simulink model "Sample156"  (Simulink 7.6)
settings: Solver=ode45  StartTime=0.0  StopTime=10.0  RelTol=1e-3
undefined symbols (not defined in the file): randint
libraries: commdigbbndfm2 x2, simulink x1, dspsrcs4 x1, commblkcod2 x1
settings Model: Creator=zhangling  LastModifiedBy=zhangling

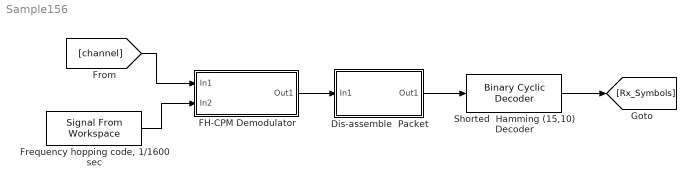
== system Sample156 ==
  Dis-assemble  Packet : Subsystem
  FH-CPM Demodulator : Subsystem
  "Frequency hopping code, 1/1600 sec" : dspsrcs4/Signal From Workspace  SystemSampleTime=-1  X=randint(1,100,78)  Ts=1/1600  nsamps=1  OutputAfterFinalValue=Cyclic repetition  ignoreOrWarnInputAndFrameLengths=off
  Shorted  Hamming (15,10) Decoder : commblkcod2/Binary Cyclic Decoder  SystemSampleTime=-1  n=7  p=4
  wires:
  [channel] -> FH-CPM Demodulator/1(In1)
  "Frequency hopping code, 1/1600 sec"/1 -> FH-CPM Demodulator/2(In2)
  Dis-assemble  Packet/1(Out1) -> Shorted  Hamming (15,10) Decoder/1
  FH-CPM Demodulator/1(Out1) -> Dis-assemble  Packet/1(In1)
  Shorted  Hamming (15,10) Decoder/1 -> [Rx_Symbols]

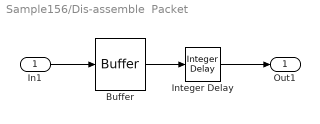
== system Sample156/Dis-assemble  Packet ==
  In1 : Inport
  Buffer : Buffer  N=15  TreatMby1Signals=One channel
  Integer Delay : simulink/Discrete/Integer Delay  NumDelays=10  vinit=0.0  samptime=-1
  Out1 : Outport
  wires:
  In1/1 -> Buffer/1
  Buffer/1 -> Integer Delay/1
  Integer Delay/1 -> Out1/1

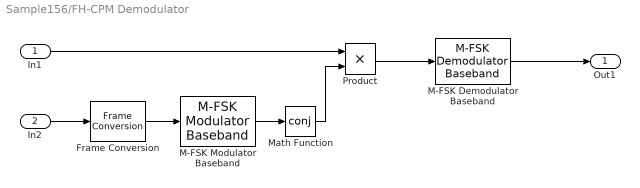
== system Sample156/FH-CPM Demodulator ==
  In1 : Inport
  In2 : Inport  Port=2
  Frame Conversion : FrameConversion
  M-FSK Demodulator Baseband : commdigbbndfm2/M-FSK Demodulator Baseband  M=2  OutType=Bit  Dec=Binary  freqSep=10  numSamp=100  RateOptions=Enforce single-rate processing  outDataType=double
  M-FSK Modulator Baseband : commdigbbndfm2/M-FSK Modulator Baseband  M=79  InType=Integer  Enc=Binary  freqSep=1e6  phaseType=Continuous  numSamp=6.25e4  RateOptions=Enforce single-rate processing  outDataType=double
  Math Function : Math  Operator=conj  SaturateOnIntegerOverflow=on
  Product : Product  RndMeth=Zero
  Out1 : Outport
  wires:
  In1/1 -> Product/1
  Product/1 -> M-FSK Demodulator Baseband/1
  In2/1 -> Frame Conversion/1
  Frame Conversion/1 -> M-FSK Modulator Baseband/1
  M-FSK Modulator Baseband/1 -> Math Function/1
  Math Function/1 -> Product/2
  M-FSK Demodulator Baseband/1 -> Out1/1
